simulink model "FPGA_UART"  (R2024a)
settings: Solver=FixedStepDiscrete  StartTime=0.0  StopTime=0.05  RelTol=1e-3
values from neighbouring files (symbols this model uses):
  Ts = 1/Fs    (= 7.50007500075e-06)    [new_generation_coeff.m]    (also in simon_test.m; simple_fft_test.m = 1/F; testPSD_c2d.m; testPSD_simulink.m)
libraries: hdlsllib x78, simulink_extras x12, simulink x5
(part 1 of 2)
settings Model: SimulationMode=accelerator  Creator=Simon  LastModifiedBy=Simon

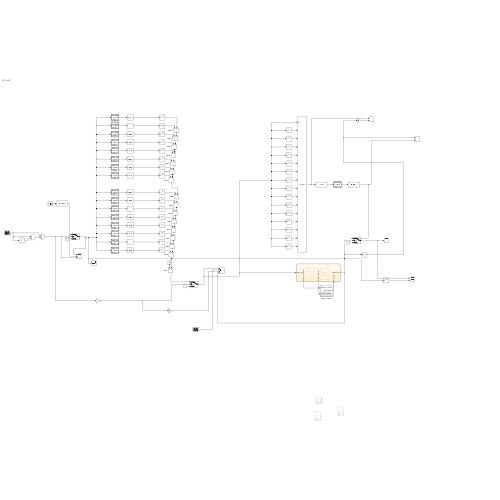
[thumbnail: Simulink's stored preview of the top-level diagram]
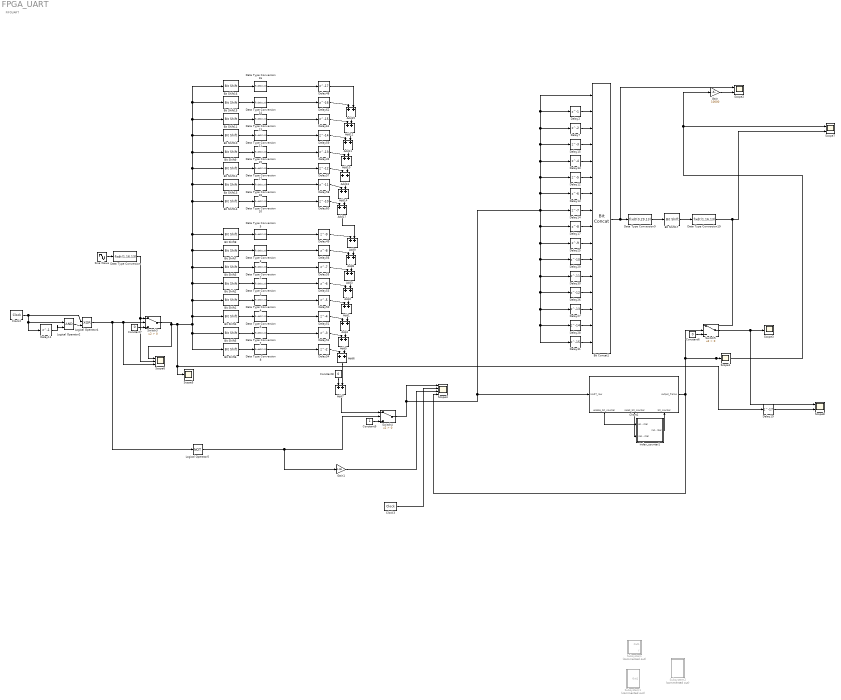
== system FPGA_UART ==
  note: FIFOUART
  Add{1..15,17} (16 alike) : Sum  OutDataTypeStr=fixdt(0,1,0)
  Bit Concat1 : hdlsllib/Logic and Bit Operations/Bit Concat  numInputs=16
  Bit Shift1 : hdlsllib/Logic and Bit Operations/Bit Shift  mode=Shift Left Logical  N=10
  Bit Shift10 : hdlsllib/Logic and Bit Operations/Bit Shift  mode=Shift Left Logical  N=1
  Bit Shift11 : hdlsllib/Logic and Bit Operations/Bit Shift  mode=Shift Right Logical  N=0
  Bit Shift12 : hdlsllib/Logic and Bit Operations/Bit Shift  mode=Shift Left Logical  N=3
  Bit Shift13 : hdlsllib/Logic and Bit Operations/Bit Shift  mode=Shift Left Logical  N=4
  Bit Shift14 : hdlsllib/Logic and Bit Operations/Bit Shift  mode=Shift Left Logical  N=5
  Bit Shift15 : hdlsllib/Logic and Bit Operations/Bit Shift  mode=Shift Right Logical  N=1
  Bit Shift16 : hdlsllib/Logic and Bit Operations/Bit Shift  mode=Shift Right Logical  N=2
  Bit Shift17 : hdlsllib/Logic and Bit Operations/Bit Shift  mode=Shift Right Logical  N=13
  Bit Shift2 : hdlsllib/Logic and Bit Operations/Bit Shift  mode=Shift Left Logical  N=9
  Bit Shift3 : hdlsllib/Logic and Bit Operations/Bit Shift  mode=Shift Left Logical  N=8
  Bit Shift4 : hdlsllib/Logic and Bit Operations/Bit Shift  mode=Shift Left Logical  N=11
  Bit Shift5 : hdlsllib/Logic and Bit Operations/Bit Shift  mode=Shift Left Logical  N=12
  Bit Shift6 : hdlsllib/Logic and Bit Operations/Bit Shift  mode=Shift Left Logical  N=13
  Bit Shift7 : hdlsllib/Logic and Bit Operations/Bit Shift  mode=Shift Left Logical  N=7
  Bit Shift8 : hdlsllib/Logic and Bit Operations/Bit Shift  mode=Shift Left Logical  N=6
  Bit Shift9 : hdlsllib/Logic and Bit Operations/Bit Shift  mode=Shift Left Logical  N=2
  Chart1 : Stateflow chart  TreatAsAtomicUnit=on
      settings: PortSchema="{\"entries\":[{\"content\":{\"sides\":[{\"content\":{\"connectorIds\":[\"In2\"]},\"type\":\"ConnectorPlacement.EquallySpacedRectSide\",\"uuid\":\"2ee02e2e-a069-4e33-9774-57cdf73b0390\"},{\"content\":{\"connectorIds\":[\"Out1\"],\"side\":\"RIGHT\"},\"type\":\"ConnectorPlacement.EquallySpacedRectSide\",\"uuid\":\"21aeb1e6-6c65-4c00-a9b7-a995856e37fb\"},{\"content\":{\"side\":\"TOP\"},\"type\":\"ConnectorPlacement.EquallySpacedRectSide\",\"uuid\":\"d38f9540-57bf-4030-828c-0c58160bc96c\"},{\"content\":{\"connectorIds\":[\"Out2\",\"Out3\",\"In1\"],\"side\":\"BOTTOM\"},\"type\":\"ConnectorPlacement.EquallySpacedRectSide\",\"uuid\":\"4fe203c5-9b79-43fe-8008-8789174ca3d6\"}]},\"type\":\"ConnectorPlacement.EquallySpacedConnector\",\"uuid\":\"11cdfd4e-ecb7-4173-8729-c2a9bb2b5432\"}],\"packageUris\":[\"http://schema.mathworks.com/mf0/Connector/R2020b\"],\"version\":\"1.0\"}"
  Clock2 : simulink_extras/Flip Flops/Clock  period=Ts*18
  Clock3 : simulink_extras/Flip Flops/Clock  period=Ts
  Constant6 : Constant  Value=0  OutDataTypeStr=fixdt(0,4,0)  SampleTime=Ts
  Constant7 : Constant  Value=0  OutDataTypeStr=fixdt(0,4,0)  SampleTime=Ts
  Constant8 : Constant  Value=0  OutDataTypeStr=fixdt(0,4,0)  SampleTime=Ts
  Constant9 : Constant  OutDataTypeStr=fixdt(0,4,0)  SampleTime=Ts
  Data Type Conversion : DataTypeConversion  OutDataTypeStr=fixdt(1,16,13)  SaturateOnIntegerOverflow=off  RndMeth=Floor
  Data Type Conversion{1..8,10..11,13..18} (16 alike) : DataTypeConversion  OutDataTypeStr=fixdt(0,1,0)  SaturateOnIntegerOverflow=off  RndMeth=Floor
  Data Type Conversion19 : DataTypeConversion  OutDataTypeStr=fixdt(1,16,13)  SaturateOnIntegerOverflow=off  RndMeth=Floor
  Data Type Conversion9 : DataTypeConversion  OutDataTypeStr=fixdt(0,29,13)  SaturateOnIntegerOverflow=off  RndMeth=Floor
  Delay11 : Delay  DelayLength=1  InitialCondition=0  SampleTime=Ts
  Delay12 : Delay  DelayLength=5  InitialCondition=0  SampleTime=Ts
  Delay13 : Delay  DelayLength=6  InitialCondition=0  SampleTime=Ts
  Delay14 : Delay  DelayLength=7  InitialCondition=0  SampleTime=Ts
  Delay15 : Delay  DelayLength=3  InitialCondition=0  SampleTime=Ts
  Delay17 : Delay  DelayLength=8  InitialCondition=0  SampleTime=Ts
  Delay19 : Delay  DelayLength=17  InitialCondition=0
  Delay2 : Delay  DelayLength=1  InitialCondition=0  SampleTime=Ts
  Delay25 : Delay  DelayLength=9  InitialCondition=0  SampleTime=Ts
  Delay26 : Delay  DelayLength=12  InitialCondition=0  SampleTime=Ts
  Delay27 : Delay  DelayLength=13  InitialCondition=0  SampleTime=Ts
  Delay28 : Delay  DelayLength=14  InitialCondition=0  SampleTime=Ts
  Delay29 : Delay  DelayLength=10  InitialCondition=0  SampleTime=Ts
  Delay30 : Delay  DelayLength=11  InitialCondition=0  SampleTime=Ts
  Delay31 : Delay  DelayLength=15  InitialCondition=0  SampleTime=Ts
  Delay32 : Delay  DelayLength=13  InitialCondition=0  SampleTime=Ts
  Delay33 : Delay  DelayLength=4  InitialCondition=0  SampleTime=Ts
  Delay48 : Delay  DelayLength=17  InitialCondition=0  SampleTime=Ts
  Delay49 : Delay  DelayLength=9  InitialCondition=0  SampleTime=Ts
  Delay50 : Delay  DelayLength=5  InitialCondition=0  SampleTime=Ts
  Delay51 : Delay  DelayLength=4  InitialCondition=0  SampleTime=Ts
  Delay52 : Delay  DelayLength=3  InitialCondition=0  SampleTime=Ts
  Delay53 : Delay  DelayLength=6  InitialCondition=0  SampleTime=Ts
  Delay54 : Delay  InitialCondition=0  SampleTime=Ts
  Delay55 : Delay  DelayLength=7  InitialCondition=0  SampleTime=Ts
  Delay56 : Delay  DelayLength=8  InitialCondition=0  SampleTime=Ts
  Delay57 : Delay  DelayLength=12  InitialCondition=0  SampleTime=Ts
  Delay58 : Delay  DelayLength=11  InitialCondition=0  SampleTime=Ts
  Delay59 : Delay  DelayLength=14  InitialCondition=0  SampleTime=Ts
  Delay60 : Delay  DelayLength=10  InitialCondition=0  SampleTime=Ts
  Delay61 : Delay  DelayLength=15  InitialCondition=0  SampleTime=Ts
  Delay62 : Delay  DelayLength=16  InitialCondition=0  SampleTime=Ts
  Delay7 : Delay  InitialCondition=0  SampleTime=Ts
  Gain : Gain  Gain=10000
  Gain1 : Gain  Gain=1.05
  Logical Operator2 : Logic  IconShape=distinctive  AllPortsSameDT=off  OutDataTypeStr=boolean
  Logical Operator4 : Logic  Operator=XOR  IconShape=distinctive  AllPortsSameDT=off  OutDataTypeStr=boolean
  Logical Operator5 : Logic  Operator=NOT  IconShape=distinctive  AllPortsSameDT=off  OutDataTypeStr=boolean
  Scope1 : Scope
  Scope2 : Scope  NumInputPorts=2
  Scope3 : Scope
  Scope4 : Scope  NumInputPorts=4
  Scope5 : Scope
  Scope6 : Scope  NumInputPorts=3
  Scope7 : Scope  NumInputPorts=2
  Scope8 : Scope  NumInputPorts=2
  Sine Wave : Sin  Amplitude=2  Frequency=1000  SampleTime=Ts*18
  Subsystem : Subsystem  Commented=on
  Subsystem1 : Subsystem  Commented=on
  Subsystem2 : Subsystem  Commented=on
  Switch3 : Switch  Criteria=u2 > Threshold  SaturateOnIntegerOverflow=off  InputSameDT=off  OutDataTypeStr=Inherit: Same as first input
  Switch4 : Switch  Criteria=u2 > Threshold  OutDataTypeStr=fixdt(0,1,0)  SaturateOnIntegerOverflow=off  InputSameDT=off
  Switch5 : Switch  Criteria=u2 > Threshold  SaturateOnIntegerOverflow=off  InputSameDT=off  OutDataTypeStr=Inherit: Same as first input
  index_counter1 : Subsystem
  wires:
  Delay19/1 -> Scope8/2
  Switch5/1 -> Scope8/1, Scope3/1
  Data Type Conversion/1 -> Scope6/2, Switch3/1
  Data Type Conversion9/1 -> Bit Shift17/1
  Bit Shift17/1 -> Data Type Conversion19/1
  Delay26/1 -> Bit Concat1/13
  Delay30/1 -> Bit Concat1/12
  Delay33/1 -> Bit Concat1/5
  Delay27/1 -> Bit Concat1/14
  Delay29/1 -> Bit Concat1/11
  Delay28/1 -> Bit Concat1/15
  Delay17/1 -> Bit Concat1/9
  Delay14/1 -> Bit Concat1/8
  Delay13/1 -> Bit Concat1/7
  Delay31/1 -> Bit Concat1/16
  Delay15/1 -> Bit Concat1/4
  Delay7/1 -> Bit Concat1/3
  Delay12/1 -> Bit Concat1/6
  Switch4/1 -> Delay31/1, Delay28/1, Delay27/1, Delay26/1, Delay30/1, Delay29/1, Delay25/1, Delay17/1, Delay14/1, Delay2/1, Bit Concat1/1, Delay7/1, Delay15/1, Delay33/1, Delay12/1, Delay13/1, Chart1/2(UART_raw), Scope4/1
  Delay25/1 -> Bit Concat1/10
  Delay2/1 -> Bit Concat1/2
  Gain/1 -> Scope2/2
  Data Type Conversion19/1 -> Scope7/2, Switch5/1
  Bit Shift6/1 -> Data Type Conversion8/1
  Add14/1 -> Add17/2
  Add17/1 -> Add9/2
  Delay60/1 -> Add17/1
  Add13/1 -> Add14/2
  Delay57/1 -> Add13/1
  Delay32/1 -> Add10/1
  Bit Shift9/1 -> Data Type Conversion15/1
  Bit Shift13/1 -> Data Type Conversion18/1
  Delay58/1 -> Add14/1
  Data Type Conversion17/1 -> Delay57/1
  Bit Shift12/1 -> Data Type Conversion17/1
  Data Type Conversion18/1 -> Delay58/1
  Data Type Conversion15/1 -> Delay32/1
  Data Type Conversion11/1 -> Delay59/1
  Bit Shift10/1 -> Data Type Conversion11/1
  Add10/1 -> Add13/2
  Delay61/1 -> Add12/1
  Bit Shift11/1 -> Data Type Conversion13/1
  Data Type Conversion13/1 -> Delay61/1
  Data Type Conversion14/1 -> Delay62/1
  Bit Shift15/1 -> Data Type Conversion14/1
  Delay62/1 -> Add15/1
  Bit Shift16/1 -> Data Type Conversion16/1
  Data Type Conversion16/1 -> Delay48/1
  Add11/1 -> Add10/2
  Delay59/1 -> Add11/1
  Add12/1 -> Add11/2
  Add15/1 -> Add12/2
  Switch3/1 -> Delay19/1, Scope5/1, Bit Shift4/1, Bit Shift1/1, Bit Shift2/1, Bit Shift3/1, Bit Shift7/1, Bit Shift8/1, Bit Shift14/1, Bit Shift13/1, Bit Shift12/1, Bit Shift9/1, Bit Shift10/1, Bit Shift11/1, Bit Shift15/1, Bit Shift16/1, Bit Shift6/1, Bit Shift5/1, Scope6/1
  Delay48/1 -> Add15/2
  Add9/1 -> Add8/2
  Bit Shift14/1 -> Data Type Conversion10/1
  Data Type Conversion10/1 -> Delay60/1
  Add8/1 -> Add3/2
  Add3/1 -> Add2/2
  Delay53/1 -> Add2/1
  Add2/1 -> Add1/2
  Data Type Conversion5/1 -> Delay49/1
  Bit Shift8/1 -> Data Type Conversion5/1
  Delay49/1 -> Add9/1
  Delay56/1 -> Add8/1
  Bit Shift7/1 -> Data Type Conversion3/1
  Data Type Conversion3/1 -> Delay56/1
  Data Type Conversion2/1 -> Delay55/1
  Bit Shift3/1 -> Data Type Conversion2/1
  Delay55/1 -> Add3/1
  Add1/1 -> Add4/2
  Bit Shift2/1 -> Data Type Conversion1/1
  Data Type Conversion1/1 -> Delay53/1
  Data Type Conversion4/1 -> Delay50/1
  Add6/1 -> Add7/2
  Data Type Conversion7/1 -> Delay52/1
  Bit Shift4/1 -> Data Type Conversion6/1
  Delay11/1 -> Logical Operator2/2
  Chart1/3(reset_bit_counter) -> index_counter1/2(reset_bit_counter)
  Constant9/1 -> Switch4/3
  Logical Operator2/1 -> Logical Operator4/2
  Constant7/1 -> Switch3/3
  Delay54/1 -> Add6/1
  Data Type Conversion6/1 -> Delay51/1
  Add5/1 -> Add6/2
  Gain1/1 -> Scope4/3
  Data Type Conversion8/1 -> Delay54/1
  Delay52/1 -> Add5/1
  Bit Shift5/1 -> Data Type Conversion7/1
  Clock3/1 -> Scope4/2
  Bit Shift1/1 -> Data Type Conversion4/1
  Sine Wave/1 -> Data Type Conversion/1
  Add7/1 -> Switch4/1
  Logical Operator5/1 -> Gain1/1, Switch4/2
  Delay50/1 -> Add1/1
  Logical Operator4/1 -> Logical Operator5/1, Scope6/3, Switch3/2
  Delay51/1 -> Add4/1
  index_counter1/1(index_counter) -> Chart1/1(bit_counter)
  Chart1/2(enable_bit_counter) -> index_counter1/1(enable_bit_counter)
  Chart1/1(output_frame) -> Scope1/1, Scope7/1, Gain/1, Switch5/2, Scope4/4
  Constant8/1 -> Add7/1
  Clock2/1 -> Delay11/1, Logical Operator2/1, Logical Operator4/1
  Add4/1 -> Add5/2
  Bit Concat1/1 -> Data Type Conversion9/1, Scope2/1
  Constant6/1 -> Switch5/3

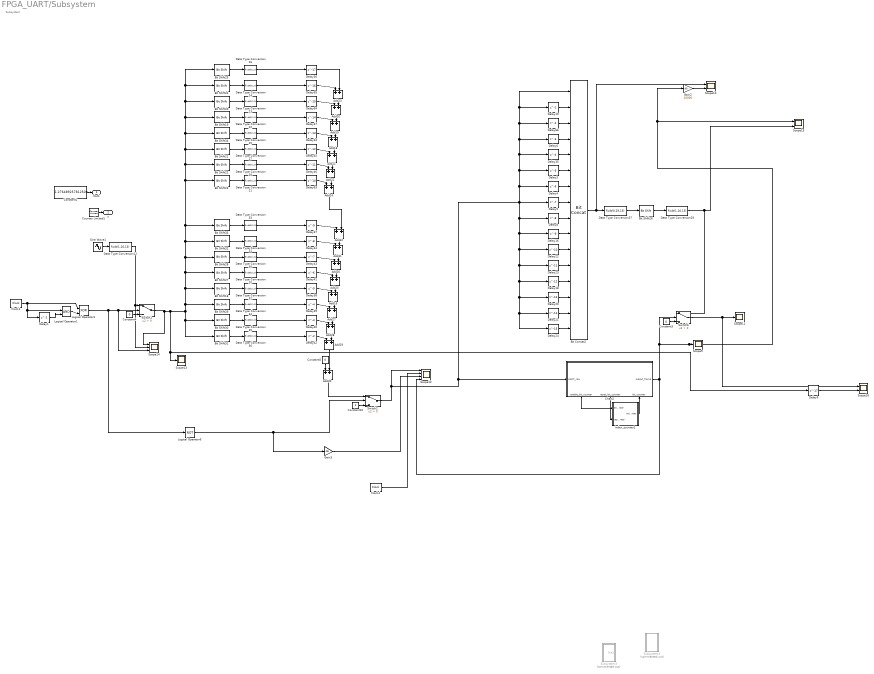
== system FPGA_UART/Subsystem ==
  note: Subsystem
  Add{16,18..32} (16 alike) : Sum  OutDataTypeStr=fixdt(0,1,0)
  Bit Concat2 : hdlsllib/Logic and Bit Operations/Bit Concat  numInputs=16
  Bit Shift18 : hdlsllib/Logic and Bit Operations/Bit Shift  mode=Shift Left Logical  N=10
  Bit Shift19 : hdlsllib/Logic and Bit Operations/Bit Shift  mode=Shift Left Logical  N=1
  Bit Shift20 : hdlsllib/Logic and Bit Operations/Bit Shift  mode=Shift Right Logical  N=0
  Bit Shift21 : hdlsllib/Logic and Bit Operations/Bit Shift  mode=Shift Left Logical  N=3
  Bit Shift22 : hdlsllib/Logic and Bit Operations/Bit Shift  mode=Shift Left Logical  N=4
  Bit Shift23 : hdlsllib/Logic and Bit Operations/Bit Shift  mode=Shift Left Logical  N=5
  Bit Shift24 : hdlsllib/Logic and Bit Operations/Bit Shift  mode=Shift Right Logical  N=1
  Bit Shift25 : hdlsllib/Logic and Bit Operations/Bit Shift  mode=Shift Right Logical  N=2
  Bit Shift26 : hdlsllib/Logic and Bit Operations/Bit Shift  mode=Shift Right Logical  N=13
  Bit Shift27 : hdlsllib/Logic and Bit Operations/Bit Shift  mode=Shift Left Logical  N=9
  Bit Shift28 : hdlsllib/Logic and Bit Operations/Bit Shift  mode=Shift Left Logical  N=8
  Bit Shift29 : hdlsllib/Logic and Bit Operations/Bit Shift  mode=Shift Left Logical  N=11
  Bit Shift30 : hdlsllib/Logic and Bit Operations/Bit Shift  mode=Shift Left Logical  N=12
  Bit Shift31 : hdlsllib/Logic and Bit Operations/Bit Shift  mode=Shift Left Logical  N=13
  Bit Shift32 : hdlsllib/Logic and Bit Operations/Bit Shift  mode=Shift Left Logical  N=7
  Bit Shift33 : hdlsllib/Logic and Bit Operations/Bit Shift  mode=Shift Left Logical  N=6
  Bit Shift34 : hdlsllib/Logic and Bit Operations/Bit Shift  mode=Shift Left Logical  N=2
  Chart2 : Stateflow chart  TreatAsAtomicUnit=on
      settings: PortSchema="{\"entries\":[{\"content\":{\"sides\":[{\"content\":{\"connectorIds\":[\"In2\"]},\"type\":\"ConnectorPlacement.EquallySpacedRectSide\",\"uuid\":\"2ee02e2e-a069-4e33-9774-57cdf73b0390\"},{\"content\":{\"connectorIds\":[\"Out1\"],\"side\":\"RIGHT\"},\"type\":\"ConnectorPlacement.EquallySpacedRectSide\",\"uuid\":\"21aeb1e6-6c65-4c00-a9b7-a995856e37fb\"},{\"content\":{\"side\":\"TOP\"},\"type\":\"ConnectorPlacement.EquallySpacedRectSide\",\"uuid\":\"d38f9540-57bf-4030-828c-0c58160bc96c\"},{\"content\":{\"connectorIds\":[\"Out2\",\"Out3\",\"In1\"],\"side\":\"BOTTOM\"},\"type\":\"ConnectorPlacement.EquallySpacedRectSide\",\"uuid\":\"4fe203c5-9b79-43fe-8008-8789174ca3d6\"}]},\"type\":\"ConnectorPlacement.EquallySpacedConnector\",\"uuid\":\"11cdfd4e-ecb7-4173-8729-c2a9bb2b5432\"}],\"packageUris\":[\"http://schema.mathworks.com/mf0/Connector/R2020b\"],\"version\":\"1.0\"}"
  Clock1 : simulink_extras/Flip Flops/Clock  period=Ts*18
  Clock4 : simulink_extras/Flip Flops/Clock  period=Ts
  Constant1 : Constant  Value=1.276489257812500  OutDataTypeStr=fixdt(1,16,13)  SampleTime=Ts
  Constant10 : Constant  OutDataTypeStr=fixdt(0,4,0)  SampleTime=Ts
  Constant3 : Constant  Value=0  OutDataTypeStr=fixdt(0,4,0)  SampleTime=Ts
  Constant4 : Constant  Value=0  OutDataTypeStr=fixdt(0,4,0)  SampleTime=Ts
  Constant5 : Constant  Value=0  OutDataTypeStr=fixdt(0,4,0)  SampleTime=Ts
  Counter Limited1 : simulink/Sources/Counter Limited  uplimit=32  tsamp=Ts*18
  Data Type Conversion12 : DataTypeConversion  OutDataTypeStr=fixdt(1,16,13)  SaturateOnIntegerOverflow=off  RndMeth=Floor
  Data Type Conversion{20..28,30..36} (16 alike) : DataTypeConversion  OutDataTypeStr=fixdt(0,1,0)  SaturateOnIntegerOverflow=off  RndMeth=Floor
  Data Type Conversion29 : DataTypeConversion  OutDataTypeStr=fixdt(1,16,13)  SaturateOnIntegerOverflow=off  RndMeth=Floor
  Data Type Conversion37 : DataTypeConversion  OutDataTypeStr=fixdt(0,29,13)  SaturateOnIntegerOverflow=off  RndMeth=Floor
  Delay1 : Delay  DelayLength=1  InitialCondition=0  SampleTime=Ts
  Delay10 : Delay  DelayLength=1  InitialCondition=0  SampleTime=Ts
  Delay16 : Delay  DelayLength=9  InitialCondition=0  SampleTime=Ts
  Delay18 : Delay  DelayLength=12  InitialCondition=0  SampleTime=Ts
  Delay20 : Delay  DelayLength=13  InitialCondition=0  SampleTime=Ts
  Delay21 : Delay  DelayLength=14  InitialCondition=0  SampleTime=Ts
  Delay22 : Delay  DelayLength=10  InitialCondition=0  SampleTime=Ts
  Delay23 : Delay  DelayLength=11  InitialCondition=0  SampleTime=Ts
  Delay24 : Delay  DelayLength=15  InitialCondition=0  SampleTime=Ts
  Delay3 : Delay  DelayLength=5  InitialCondition=0  SampleTime=Ts
  Delay34 : Delay  DelayLength=13  InitialCondition=0  SampleTime=Ts
  Delay35 : Delay  DelayLength=4  InitialCondition=0  SampleTime=Ts
  Delay36 : Delay  DelayLength=17  InitialCondition=0  SampleTime=Ts
  Delay37 : Delay  DelayLength=9  InitialCondition=0  SampleTime=Ts
  Delay38 : Delay  DelayLength=5  InitialCondition=0  SampleTime=Ts
  Delay39 : Delay  DelayLength=4  InitialCondition=0  SampleTime=Ts
  Delay4 : Delay  DelayLength=6  InitialCondition=0  SampleTime=Ts
  Delay40 : Delay  DelayLength=3  InitialCondition=0  SampleTime=Ts
  Delay41 : Delay  DelayLength=6  InitialCondition=0  SampleTime=Ts
  Delay42 : Delay  InitialCondition=0  SampleTime=Ts
  Delay43 : Delay  DelayLength=7  InitialCondition=0  SampleTime=Ts
  Delay44 : Delay  DelayLength=8  InitialCondition=0  SampleTime=Ts
  Delay45 : Delay  DelayLength=12  InitialCondition=0  SampleTime=Ts
  Delay46 : Delay  DelayLength=11  InitialCondition=0  SampleTime=Ts
  Delay47 : Delay  DelayLength=14  InitialCondition=0  SampleTime=Ts
  Delay5 : Delay  DelayLength=7  InitialCondition=0  SampleTime=Ts
  Delay6 : Delay  DelayLength=3  InitialCondition=0  SampleTime=Ts
  Delay63 : Delay  DelayLength=10  InitialCondition=0  SampleTime=Ts
  Delay64 : Delay  DelayLength=15  InitialCondition=0  SampleTime=Ts
  Delay65 : Delay  DelayLength=16  InitialCondition=0  SampleTime=Ts
  Delay66 : Delay  InitialCondition=0  SampleTime=Ts
  Delay8 : Delay  DelayLength=8  InitialCondition=0  SampleTime=Ts
  Delay9 : Delay  DelayLength=17  InitialCondition=0
  Gain2 : Gain  Gain=10000
  Gain3 : Gain  Gain=1.05
  Logical Operator1 : Logic  IconShape=distinctive  AllPortsSameDT=off  OutDataTypeStr=boolean
  Logical Operator3 : Logic  Operator=XOR  IconShape=distinctive  AllPortsSameDT=off  OutDataTypeStr=boolean
  Logical Operator6 : Logic  Operator=NOT  IconShape=distinctive  AllPortsSameDT=off  OutDataTypeStr=boolean
  Scope10 : Scope  NumInputPorts=2
  Scope11 : Scope
  Scope12 : Scope  NumInputPorts=4
  Scope13 : Scope
  Scope14 : Scope  NumInputPorts=3
  Scope15 : Scope  NumInputPorts=2
  Scope16 : Scope  NumInputPorts=2
  Scope9 : Scope
  Sine Wave1 : Sin  Amplitude=2  Frequency=1000  SampleTime=Ts*18
  Subsystem3 : Subsystem  Commented=on
  Subsystem4 : Subsystem  Commented=on
  Switch1 : Switch  Criteria=u2 > Threshold  SaturateOnIntegerOverflow=off  InputSameDT=off  OutDataTypeStr=Inherit: Same as first input
  Switch2 : Switch  Criteria=u2 > Threshold  OutDataTypeStr=fixdt(0,1,0)  SaturateOnIntegerOverflow=off  InputSameDT=off
  Switch6 : Switch  Criteria=u2 > Threshold  SaturateOnIntegerOverflow=off  InputSameDT=off  OutDataTypeStr=Inherit: Same as first input
  index_counter2 : Subsystem
  Out1 : Outport
  y : Outport  Port=2
  wires:
  Add23/1 -> Add20/2
  Add27/1 -> Add28/2
  Switch2/1 -> Delay24/1, Delay21/1, Delay20/1, Delay18/1, Delay23/1, Delay22/1, Delay16/1, Delay8/1, Delay5/1, Delay10/1, Bit Concat2/1, Delay66/1, Delay6/1, Delay35/1, Delay3/1, Delay4/1, Chart2/2(UART_raw), Scope12/1
  Switch1/1 -> Delay9/1, Scope13/1, Bit Shift29/1, Bit Shift18/1, Bit Shift27/1, Bit Shift28/1, Bit Shift32/1, Bit Shift33/1, Bit Shift23/1, Bit Shift22/1, Bit Shift21/1, Bit Shift34/1, Bit Shift19/1, Bit Shift20/1, Bit Shift24/1, Bit Shift25/1, Bit Shift31/1, Bit Shift30/1, Scope14/1
  Add25/1 -> Add16/2
  Clock1/1 -> Delay1/1, Logical Operator1/1, Logical Operator3/1
  Delay66/1 -> Bit Concat2/3
  Logical Operator3/1 -> Logical Operator6/1, Scope14/3, Switch1/2
  Delay38/1 -> Add16/1
  Delay44/1 -> Add31/1
  Delay37/1 -> Add32/1
  Add30/1 -> Switch2/1
  Delay22/1 -> Bit Concat2/11
  Add21/1 -> Add22/2
  Clock4/1 -> Scope12/2
  Add31/1 -> Add26/2
  Delay65/1 -> Add23/1
  Bit Shift19/1 -> Data Type Conversion22/1
  Delay36/1 -> Add23/2
  Bit Shift21/1 -> Data Type Conversion27/1
  Constant4/1 -> Switch1/3
  Bit Shift23/1 -> Data Type Conversion21/1
  Delay42/1 -> Add29/1
  Data Type Conversion27/1 -> Delay45/1
  Delay35/1 -> Bit Concat2/5
  Data Type Conversion31/1 -> Delay44/1
  Add28/1 -> Add29/2
  Bit Shift33/1 -> Data Type Conversion33/1
  Add22/1 -> Add24/2
  Switch6/1 -> Scope16/1, Scope11/1
  Add20/1 -> Add19/2
  Data Type Conversion29/1 -> Scope15/2, Switch6/1
  Delay6/1 -> Bit Concat2/4
  Delay16/1 -> Bit Concat2/10
  Add24/1 -> Add32/2
  Bit Shift27/1 -> Data Type Conversion20/1
  Chart2/1(output_frame) -> Scope9/1, Scope15/1, Gain2/1, Switch6/2, Scope12/4
  Add32/1 -> Add31/2
  Delay47/1 -> Add19/1
  Gain3/1 -> Scope12/3
  Data Type Conversion21/1 -> Delay63/1
  Delay34/1 -> Add18/1
  Data Type Conversion23/1 -> Delay64/1
  Bit Shift20/1 -> Data Type Conversion23/1
  Add19/1 -> Add18/2
  Data Type Conversion22/1 -> Delay47/1
  Constant5/1 -> Add30/1
  Data Type Conversion24/1 -> Delay65/1
  Bit Shift34/1 -> Data Type Conversion25/1
  Add18/1 -> Add21/2
  Delay20/1 -> Bit Concat2/14
  Data Type Conversion25/1 -> Delay34/1
  Delay64/1 -> Add20/1
  Data Type Conversion26/1 -> Delay36/1
  Bit Shift24/1 -> Data Type Conversion24/1
  Data Type Conversion20/1 -> Delay41/1
  Delay43/1 -> Add26/1
  Delay41/1 -> Add25/1
  Bit Shift25/1 -> Data Type Conversion26/1
  Bit Shift32/1 -> Data Type Conversion31/1
  Constant3/1 -> Switch6/3
  Data Type Conversion12/1 -> Scope14/2, Switch1/1
  Data Type Conversion28/1 -> Delay46/1
  Constant1/1 -> Out1/1
  Bit Shift22/1 -> Data Type Conversion28/1
  Data Type Conversion30/1 -> Delay43/1
  Delay46/1 -> Add22/1
  Data Type Conversion33/1 -> Delay37/1
  Data Type Conversion34/1 -> Delay39/1
  Logical Operator1/1 -> Logical Operator3/2
  Bit Shift28/1 -> Data Type Conversion30/1
  Add16/1 -> Add27/2
  Delay24/1 -> Bit Concat2/16
  Delay5/1 -> Bit Concat2/8
  Data Type Conversion32/1 -> Delay38/1
  Delay18/1 -> Bit Concat2/13
  Bit Shift26/1 -> Data Type Conversion29/1
  Bit Shift31/1 -> Data Type Conversion36/1
  Data Type Conversion37/1 -> Bit Shift26/1
  Delay9/1 -> Scope16/2
  Sine Wave1/1 -> Data Type Conversion12/1
  Chart2/2(enable_bit_counter) -> index_counter2/1(enable_bit_counter)
  Delay21/1 -> Bit Concat2/15
  Delay8/1 -> Bit Concat2/9
  Delay1/1 -> Logical Operator1/2
  Delay4/1 -> Bit Concat2/7
  Delay23/1 -> Bit Concat2/12
  index_counter2/1(index_counter) -> Chart2/1(bit_counter)
  Chart2/3(reset_bit_counter) -> index_counter2/2(reset_bit_counter)
  Delay39/1 -> Add27/1
  Data Type Conversion35/1 -> Delay40/1
  Bit Concat2/1 -> Data Type Conversion37/1, Scope10/1
  Constant10/1 -> Switch2/3
  Logical Operator6/1 -> Gain3/1, Switch2/2
  Add29/1 -> Add30/2
  Delay3/1 -> Bit Concat2/6
  Bit Shift29/1 -> Data Type Conversion34/1
  Bit Shift30/1 -> Data Type Conversion35/1
  Data Type Conversion36/1 -> Delay42/1
  Bit Shift18/1 -> Data Type Conversion32/1
  Delay40/1 -> Add28/1
  Add26/1 -> Add25/2
  Counter Limited1/1 -> y/1
  Delay45/1 -> Add21/1
  Delay63/1 -> Add24/1
  Gain2/1 -> Scope10/2
  Delay10/1 -> Bit Concat2/2

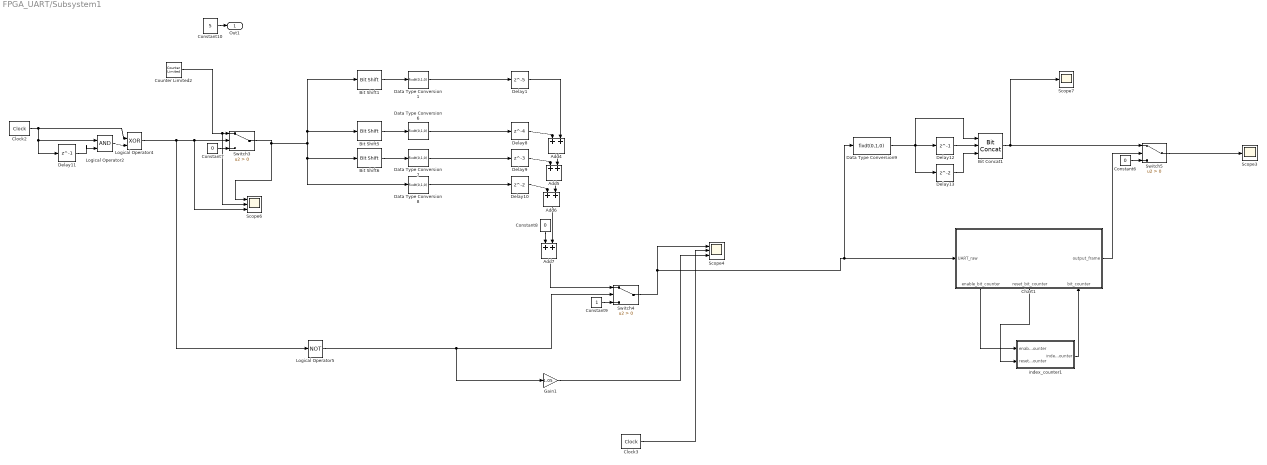
== system FPGA_UART/Subsystem1 ==
  Add{4..7} (4 alike) : Sum
  Bit Concat1 : hdlsllib/Logic and Bit Operations/Bit Concat  numInputs=3
  Bit Shift1 : hdlsllib/Logic and Bit Operations/Bit Shift  mode=Shift Right Logical  N=3
  Bit Shift5 : hdlsllib/Logic and Bit Operations/Bit Shift  mode=Shift Right Logical  N=2
  Bit Shift6 : hdlsllib/Logic and Bit Operations/Bit Shift  mode=Shift Right Logical  N=1
  Chart1 : Stateflow chart  TreatAsAtomicUnit=on
      settings: PortSchema="{\"entries\":[{\"content\":{\"sides\":[{\"content\":{\"connectorIds\":[\"In2\"]},\"type\":\"ConnectorPlacement.EquallySpacedRectSide\",\"uuid\":\"2ee02e2e-a069-4e33-9774-57cdf73b0390\"},{\"content\":{\"connectorIds\":[\"Out1\"],\"side\":\"RIGHT\"},\"type\":\"ConnectorPlacement.EquallySpacedRectSide\",\"uuid\":\"21aeb1e6-6c65-4c00-a9b7-a995856e37fb\"},{\"content\":{\"side\":\"TOP\"},\"type\":\"ConnectorPlacement.EquallySpacedRectSide\",\"uuid\":\"d38f9540-57bf-4030-828c-0c58160bc96c\"},{\"content\":{\"connectorIds\":[\"Out2\",\"Out3\",\"In1\"],\"side\":\"BOTTOM\"},\"type\":\"ConnectorPlacement.EquallySpacedRectSide\",\"uuid\":\"4fe203c5-9b79-43fe-8008-8789174ca3d6\"}]},\"type\":\"ConnectorPlacement.EquallySpacedConnector\",\"uuid\":\"11cdfd4e-ecb7-4173-8729-c2a9bb2b5432\"}],\"packageUris\":[\"http://schema.mathworks.com/mf0/Connector/R2020b\"],\"version\":\"1.0\"}"
  Clock2 : simulink_extras/Flip Flops/Clock  period=Ts*6
  Clock3 : simulink_extras/Flip Flops/Clock  period=Ts
  Constant10 : Constant  Value=5  OutDataTypeStr=fixdt(0,4,0)  SampleTime=Ts*5
  Constant6 : Constant  Value=0  OutDataTypeStr=fixdt(0,4,0)  SampleTime=Ts
  Constant7 : Constant  Value=0  OutDataTypeStr=fixdt(0,4,0)  SampleTime=Ts
  Constant8 : Constant  Value=0  OutDataTypeStr=fixdt(0,4,0)  SampleTime=Ts
  Constant9 : Constant  OutDataTypeStr=fixdt(0,4,0)  SampleTime=Ts
  Counter Limited2 : simulink/Sources/Counter Limited  uplimit=7  tsamp=Ts*6
  Data Type Conversion{1,6..8} (4 alike) : DataTypeConversion  OutDataTypeStr=fixdt(0,1,0)  SaturateOnIntegerOverflow=off  RndMeth=Floor
  Data Type Conversion9 : DataTypeConversion  OutDataTypeStr=fixdt(0,1,0)  RndMeth=Floor
  Delay1 : Delay  DelayLength=5  InitialCondition=0  SampleTime=Ts
  Delay10 : Delay  InitialCondition=0  SampleTime=Ts
  Delay11 : Delay  DelayLength=1  InitialCondition=0  SampleTime=Ts
  Delay12 : Delay  DelayLength=1  InitialCondition=0  SampleTime=Ts
  Delay13 : Delay  InitialCondition=0  SampleTime=Ts
  Delay8 : Delay  DelayLength=4  InitialCondition=0  SampleTime=Ts
  Delay9 : Delay  DelayLength=3  InitialCondition=0  SampleTime=Ts
  Gain1 : Gain  Gain=1.05
  Logical Operator2 : Logic  IconShape=distinctive  AllPortsSameDT=off  OutDataTypeStr=boolean
  Logical Operator4 : Logic  Operator=XOR  IconShape=distinctive  AllPortsSameDT=off  OutDataTypeStr=boolean
  Logical Operator5 : Logic  Operator=NOT  IconShape=distinctive  AllPortsSameDT=off  OutDataTypeStr=boolean
  Scope3 : Scope
  Scope4 : Scope  NumInputPorts=3
  Scope6 : Scope  NumInputPorts=3
  Scope7 : Scope
  Switch3 : Switch  Criteria=u2 > Threshold  SaturateOnIntegerOverflow=off  InputSameDT=off
  Switch4 : Switch  Criteria=u2 > Threshold  SaturateOnIntegerOverflow=off  InputSameDT=off
  Switch5 : Switch  Criteria=u2 > Threshold  OutDataTypeStr=fixdt(0,3,0)  SaturateOnIntegerOverflow=off  InputSameDT=off
  index_counter1 : Subsystem
  Out1 : Outport
  wires:
  Add6/1 -> Add7/2
  Data Type Conversion7/1 -> Delay9/1
  Bit Shift5/1 -> Data Type Conversion6/1
  Delay11/1 -> Logical Operator2/2
  Chart1/3(reset_bit_counter) -> index_counter1/2(reset_bit_counter)
  Constant9/1 -> Switch4/3
  Logical Operator2/1 -> Logical Operator4/2
  Constant7/1 -> Switch3/3
  Delay10/1 -> Add6/1
  Data Type Conversion6/1 -> Delay8/1
  Delay12/1 -> Bit Concat1/2
  Add5/1 -> Add6/2
  Gain1/1 -> Scope4/3
  Switch5/1 -> Scope3/1
  Data Type Conversion8/1 -> Delay10/1
  Delay9/1 -> Add5/1
  Delay13/1 -> Bit Concat1/3
  Bit Shift6/1 -> Data Type Conversion7/1
  Clock3/1 -> Scope4/2
  Counter Limited2/1 -> Switch3/1, Scope6/2
  Add7/1 -> Switch4/1
  Constant10/1 -> Out1/1
  Logical Operator5/1 -> Switch4/2, Gain1/1
  Logical Operator4/1 -> Switch3/2, Scope6/3, Logical Operator5/1
  Data Type Conversion9/1 -> Delay12/1, Delay13/1, Bit Concat1/1
  Delay8/1 -> Add4/1
  index_counter1/1(index_counter) -> Chart1/1(bit_counter)
  Chart1/2(enable_bit_counter) -> index_counter1/1(enable_bit_counter)
  Switch4/1 -> Scope4/1, Data Type Conversion9/1, Chart1/2(UART_raw)
  Chart1/1(output_frame) -> Switch5/2
  Constant8/1 -> Add7/1
  Clock2/1 -> Logical Operator4/1, Logical Operator2/1, Delay11/1
  Add4/1 -> Add5/2
  Bit Concat1/1 -> Scope7/1, Switch5/1
  Constant6/1 -> Switch5/3
  Delay1/1 -> Add4/2
  Switch3/1 -> Scope6/1, Bit Shift6/1, Data Type Conversion8/1, Bit Shift1/1, Bit Shift5/1
  Data Type Conversion1/1 -> Delay1/1
  Bit Shift1/1 -> Data Type Conversion1/1

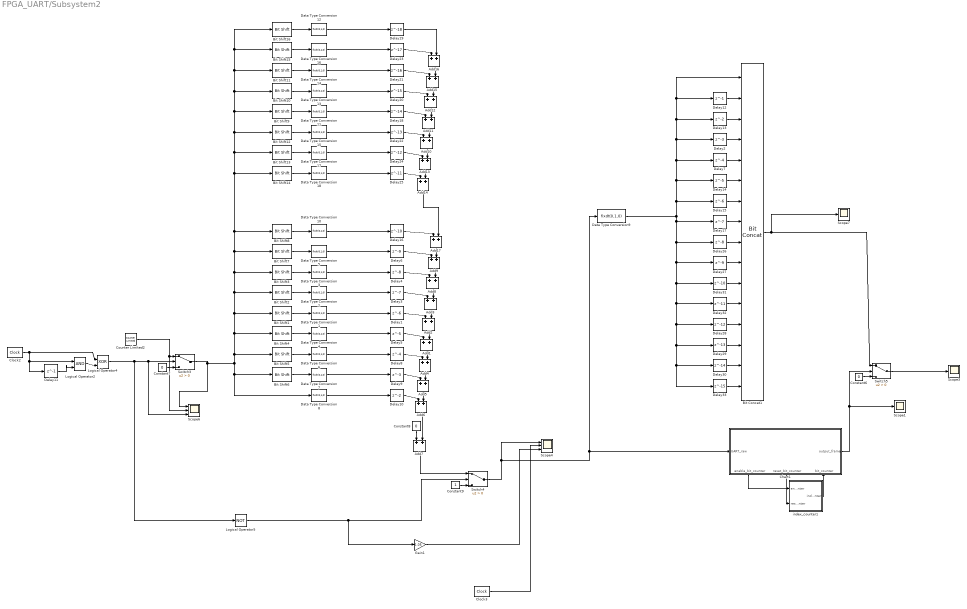
== system FPGA_UART/Subsystem2 ==
  Add{1..17} (17 alike) : Sum
  Bit Concat1 : hdlsllib/Logic and Bit Operations/Bit Concat  numInputs=16
  Bit Shift1 : hdlsllib/Logic and Bit Operations/Bit Shift  mode=Shift Right Logical  N=4
  Bit Shift10 : hdlsllib/Logic and Bit Operations/Bit Shift  mode=Shift Right Logical  N=13
  Bit Shift11 : hdlsllib/Logic and Bit Operations/Bit Shift  mode=Shift Right Logical  N=14
  Bit Shift12 : hdlsllib/Logic and Bit Operations/Bit Shift  mode=Shift Right Logical  N=11
  Bit Shift13 : hdlsllib/Logic and Bit Operations/Bit Shift  mode=Shift Right Logical  N=10
  Bit Shift14 : hdlsllib/Logic and Bit Operations/Bit Shift  mode=Shift Right Logical  N=9
  Bit Shift15 : hdlsllib/Logic and Bit Operations/Bit Shift  mode=Shift Right Logical  N=15
  Bit Shift16 : hdlsllib/Logic and Bit Operations/Bit Shift  mode=Shift Right Logical  N=16
  Bit Shift2 : hdlsllib/Logic and Bit Operations/Bit Shift  mode=Shift Right Logical  N=5
  Bit Shift3 : hdlsllib/Logic and Bit Operations/Bit Shift  mode=Shift Right Logical  N=6
  Bit Shift4 : hdlsllib/Logic and Bit Operations/Bit Shift  mode=Shift Right Logical  N=3
  Bit Shift5 : hdlsllib/Logic and Bit Operations/Bit Shift  mode=Shift Right Logical  N=2
  Bit Shift6 : hdlsllib/Logic and Bit Operations/Bit Shift  mode=Shift Right Logical  N=1
  Bit Shift7 : hdlsllib/Logic and Bit Operations/Bit Shift  mode=Shift Right Logical  N=7
  Bit Shift8 : hdlsllib/Logic and Bit Operations/Bit Shift  mode=Shift Right Logical  N=8
  Bit Shift9 : hdlsllib/Logic and Bit Operations/Bit Shift  mode=Shift Right Logical  N=12
  Chart1 : Stateflow chart  TreatAsAtomicUnit=on
      settings: PortSchema="{\"entries\":[{\"content\":{\"sides\":[{\"content\":{\"connectorIds\":[\"In2\"]},\"type\":\"ConnectorPlacement.EquallySpacedRectSide\",\"uuid\":\"2ee02e2e-a069-4e33-9774-57cdf73b0390\"},{\"content\":{\"connectorIds\":[\"Out1\"],\"side\":\"RIGHT\"},\"type\":\"ConnectorPlacement.EquallySpacedRectSide\",\"uuid\":\"21aeb1e6-6c65-4c00-a9b7-a995856e37fb\"},{\"content\":{\"side\":\"TOP\"},\"type\":\"ConnectorPlacement.EquallySpacedRectSide\",\"uuid\":\"d38f9540-57bf-4030-828c-0c58160bc96c\"},{\"content\":{\"connectorIds\":[\"Out2\",\"Out3\",\"In1\"],\"side\":\"BOTTOM\"},\"type\":\"ConnectorPlacement.EquallySpacedRectSide\",\"uuid\":\"4fe203c5-9b79-43fe-8008-8789174ca3d6\"}]},\"type\":\"ConnectorPlacement.EquallySpacedConnector\",\"uuid\":\"11cdfd4e-ecb7-4173-8729-c2a9bb2b5432\"}],\"packageUris\":[\"http://schema.mathworks.com/mf0/Connector/R2020b\"],\"version\":\"1.0\"}"
  Clock2 : simulink_extras/Flip Flops/Clock  period=Ts*18
  Clock3 : simulink_extras/Flip Flops/Clock  period=Ts
  Constant6 : Constant  Value=0  OutDataTypeStr=fixdt(0,4,0)  SampleTime=Ts
  Constant7 : Constant  Value=0  OutDataTypeStr=fixdt(0,4,0)  SampleTime=Ts
  Constant8 : Constant  Value=0  OutDataTypeStr=fixdt(0,4,0)  SampleTime=Ts
  Constant9 : Constant  OutDataTypeStr=fixdt(0,4,0)  SampleTime=Ts
  Counter Limited2 : simulink/Sources/Counter Limited  uplimit=65535  tsamp=Ts*18
  Data Type Conversion{1..8,10..18} (17 alike) : DataTypeConversion  OutDataTypeStr=fixdt(0,1,0)  SaturateOnIntegerOverflow=off  RndMeth=Floor
  Data Type Conversion9 : DataTypeConversion  OutDataTypeStr=fixdt(0,1,0)  RndMeth=Floor
  Delay1 : Delay  DelayLength=6  InitialCondition=0  SampleTime=Ts
  Delay10 : Delay  InitialCondition=0  SampleTime=Ts
  Delay11 : Delay  DelayLength=1  InitialCondition=0  SampleTime=Ts
  Delay12 : Delay  DelayLength=1  InitialCondition=0  SampleTime=Ts
  Delay13 : Delay  InitialCondition=0  SampleTime=Ts
  Delay14 : Delay  DelayLength=5  InitialCondition=0  SampleTime=Ts
  Delay15 : Delay  DelayLength=6  InitialCondition=0  SampleTime=Ts
  Delay16 : Delay  DelayLength=10  InitialCondition=0  SampleTime=Ts
  Delay17 : Delay  DelayLength=7  InitialCondition=0  SampleTime=Ts
  Delay18 : Delay  DelayLength=14  InitialCondition=0  SampleTime=Ts
  Delay19 : Delay  DelayLength=18  InitialCondition=0  SampleTime=Ts
  Delay2 : Delay  DelayLength=3  InitialCondition=0  SampleTime=Ts
  Delay20 : Delay  DelayLength=15  InitialCondition=0  SampleTime=Ts
  Delay21 : Delay  DelayLength=16  InitialCondition=0  SampleTime=Ts
  Delay22 : Delay  DelayLength=13  InitialCondition=0  SampleTime=Ts
  Delay23 : Delay  DelayLength=17  InitialCondition=0  SampleTime=Ts
  Delay24 : Delay  DelayLength=12  InitialCondition=0  SampleTime=Ts
  Delay25 : Delay  DelayLength=11  InitialCondition=0  SampleTime=Ts
  Delay26 : Delay  DelayLength=8  InitialCondition=0  SampleTime=Ts
  Delay27 : Delay  DelayLength=9  InitialCondition=0  SampleTime=Ts
  Delay28 : Delay  DelayLength=12  InitialCondition=0  SampleTime=Ts
  Delay29 : Delay  DelayLength=13  InitialCondition=0  SampleTime=Ts
  Delay3 : Delay  DelayLength=7  InitialCondition=0  SampleTime=Ts
  Delay30 : Delay  DelayLength=14  InitialCondition=0  SampleTime=Ts
  Delay31 : Delay  DelayLength=10  InitialCondition=0  SampleTime=Ts
  Delay32 : Delay  DelayLength=11  InitialCondition=0  SampleTime=Ts
  Delay33 : Delay  DelayLength=15  InitialCondition=0  SampleTime=Ts
  Delay4 : Delay  DelayLength=8  InitialCondition=0  SampleTime=Ts
  Delay5 : Delay  DelayLength=5  InitialCondition=0  SampleTime=Ts
  Delay6 : Delay  DelayLength=9  InitialCondition=0  SampleTime=Ts
  Delay7 : Delay  DelayLength=4  InitialCondition=0  SampleTime=Ts
  Delay8 : Delay  DelayLength=4  InitialCondition=0  SampleTime=Ts
  Delay9 : Delay  DelayLength=3  InitialCondition=0  SampleTime=Ts
  Gain1 : Gain  Gain=1.05
  Logical Operator2 : Logic  IconShape=distinctive  AllPortsSameDT=off  OutDataTypeStr=boolean
  Logical Operator4 : Logic  Operator=XOR  IconShape=distinctive  AllPortsSameDT=off  OutDataTypeStr=boolean
  Logical Operator5 : Logic  Operator=NOT  IconShape=distinctive  AllPortsSameDT=off  OutDataTypeStr=boolean
  Scope1 : Scope
  Scope3 : Scope
  Scope4 : Scope  NumInputPorts=3
  Scope6 : Scope  NumInputPorts=3
  Scope7 : Scope
  Switch3 : Switch  Criteria=u2 > Threshold  SaturateOnIntegerOverflow=off  InputSameDT=off
  Switch4 : Switch  Criteria=u2 > Threshold  SaturateOnIntegerOverflow=off  InputSameDT=off
  Switch5 : Switch  Criteria=u2 > Threshold  SaturateOnIntegerOverflow=off  InputSameDT=off  OutDataTypeStr=Inherit: Same as first input
  index_counter1 : Subsystem
  wires:
  Delay26/1 -> Bit Concat1/9
  Delay27/1 -> Bit Concat1/10
  Delay31/1 -> Bit Concat1/11
  Delay32/1 -> Bit Concat1/12
  Delay28/1 -> Bit Concat1/13
  Delay29/1 -> Bit Concat1/14
  Delay30/1 -> Bit Concat1/15
  Delay33/1 -> Bit Concat1/16
  Delay17/1 -> Bit Concat1/8
  Delay15/1 -> Bit Concat1/7
  Delay14/1 -> Bit Concat1/6
  Delay7/1 -> Bit Concat1/5
  Delay2/1 -> Bit Concat1/4
  Delay13/1 -> Bit Concat1/3
  Delay12/1 -> Bit Concat1/2
  Add14/1 -> Add17/2
  Add17/1 -> Add9/2
  Delay16/1 -> Add17/1
  Add13/1 -> Add14/2
  Delay24/1 -> Add13/1
  Delay22/1 -> Add10/1
  Bit Shift12/1 -> Data Type Conversion15/1
  Bit Shift14/1 -> Data Type Conversion18/1
  Delay25/1 -> Add14/1
  Data Type Conversion17/1 -> Delay24/1
  Bit Shift13/1 -> Data Type Conversion17/1
  Data Type Conversion18/1 -> Delay25/1
  Data Type Conversion15/1 -> Delay22/1
  Data Type Conversion11/1 -> Delay18/1
  Bit Shift9/1 -> Data Type Conversion11/1
  Add10/1 -> Add13/2
  Delay20/1 -> Add12/1
  Bit Shift10/1 -> Data Type Conversion13/1
  Data Type Conversion13/1 -> Delay20/1
  Data Type Conversion14/1 -> Delay21/1
  Bit Shift11/1 -> Data Type Conversion14/1
  Delay21/1 -> Add15/1
  Delay23/1 -> Add16/1
  Bit Shift15/1 -> Data Type Conversion16/1
  Data Type Conversion16/1 -> Delay23/1
  Add11/1 -> Add10/2
  Delay18/1 -> Add11/1
  Add12/1 -> Add11/2
  Add15/1 -> Add12/2
  Data Type Conversion12/1 -> Delay19/1
  Switch3/1 -> Scope6/1, Bit Shift6/1, Data Type Conversion8/1, Bit Shift5/1, Bit Shift4/1, Bit Shift1/1, Bit Shift2/1, Bit Shift3/1, Bit Shift7/1, Bit Shift8/1, Bit Shift14/1, Bit Shift13/1, Bit Shift12/1, Bit Shift9/1, Bit Shift10/1, Bit Shift11/1, Bit Shift16/1, Bit Shift15/1
  Bit Shift16/1 -> Data Type Conversion12/1
  Add16/1 -> Add15/2
  Delay19/1 -> Add16/2
  Data Type Conversion9/1 -> Delay15/1, Delay14/1, Delay7/1, Delay2/1, Delay13/1, Bit Concat1/1, Delay12/1, Delay17/1, Delay26/1, Delay27/1, Delay31/1, Delay32/1, Delay28/1, Delay29/1, Delay30/1, Delay33/1
  Add9/1 -> Add8/2
  Bit Shift8/1 -> Data Type Conversion10/1
  Data Type Conversion10/1 -> Delay16/1
  Add8/1 -> Add3/2
  Add3/1 -> Add2/2
  Delay1/1 -> Add2/1
  Add2/1 -> Add1/2
  Data Type Conversion5/1 -> Delay6/1
  Bit Shift7/1 -> Data Type Conversion5/1
  Delay6/1 -> Add9/1
  Delay4/1 -> Add8/1
  Bit Shift3/1 -> Data Type Conversion3/1
  Data Type Conversion3/1 -> Delay4/1
  Data Type Conversion2/1 -> Delay3/1
  Bit Shift2/1 -> Data Type Conversion2/1
  Delay3/1 -> Add3/1
  Add1/1 -> Add4/2
  Bit Shift1/1 -> Data Type Conversion1/1
  Data Type Conversion1/1 -> Delay1/1
  Data Type Conversion4/1 -> Delay5/1
  Add6/1 -> Add7/2
  Data Type Conversion7/1 -> Delay9/1
  Bit Shift5/1 -> Data Type Conversion6/1
  Delay11/1 -> Logical Operator2/2
  Chart1/3(reset_bit_counter) -> index_counter1/2(reset_bit_counter)
  Constant9/1 -> Switch4/3
  Logical Operator2/1 -> Logical Operator4/2
  Constant7/1 -> Switch3/3
  Delay10/1 -> Add6/1
  Data Type Conversion6/1 -> Delay8/1
  Add5/1 -> Add6/2
  Gain1/1 -> Scope4/3
  Switch5/1 -> Scope3/1
  Data Type Conversion8/1 -> Delay10/1
  Delay9/1 -> Add5/1
  Bit Shift6/1 -> Data Type Conversion7/1
  Clock3/1 -> Scope4/2
  Bit Shift4/1 -> Data Type Conversion4/1
  Counter Limited2/1 -> Switch3/1, Scope6/2
  Add7/1 -> Switch4/1
  Logical Operator5/1 -> Switch4/2, Gain1/1
  Delay5/1 -> Add1/1
  Logical Operator4/1 -> Switch3/2, Scope6/3, Logical Operator5/1
  Delay8/1 -> Add4/1
  index_counter1/1(index_counter) -> Chart1/1(bit_counter)
  Chart1/2(enable_bit_counter) -> index_counter1/1(enable_bit_counter)
  Switch4/1 -> Scope4/1, Data Type Conversion9/1, Chart1/2(UART_raw)
  Chart1/1(output_frame) -> Switch5/2, Scope1/1
  Constant8/1 -> Add7/1
  Clock2/1 -> Logical Operator4/1, Logical Operator2/1, Delay11/1
  Add4/1 -> Add5/2
  Bit Concat1/1 -> Switch5/1, Scope7/1
  Constant6/1 -> Switch5/3

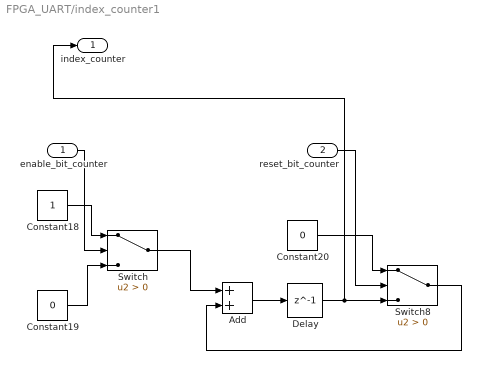
== system FPGA_UART/index_counter1 ==
  enable_bit_counter : Inport
  reset_bit_counter : Inport  Port=2
  Add : Sum  OutDataTypeStr=Inherit: Same as first input
  Constant18 : Constant  OutDataTypeStr=fixdt(0,8,0)  SampleTime=Ts
  Constant19 : Constant  Value=0  OutDataTypeStr=fixdt(0,8,0)  SampleTime=Ts
  Constant20 : Constant  Value=0  OutDataTypeStr=fixdt(0,8,0)  SampleTime=Ts
  Delay : Delay  DelayLength=1  InitialCondition=0  SampleTime=Ts
  Switch : Switch  Criteria=u2 > Threshold  SaturateOnIntegerOverflow=off  InputSameDT=off  OutDataTypeStr=Inherit: Same as first input
  Switch8 : Switch  Criteria=u2 > Threshold  SaturateOnIntegerOverflow=off  InputSameDT=off  OutDataTypeStr=Inherit: Same as first input
  index_counter : Outport
  wires:
  Constant19/1 -> Switch/3
  Switch8/1 -> Add/2
  Switch/1 -> Add/1
  Delay/1 -> index_counter/1, Switch8/3
  reset_bit_counter/1 -> Switch8/2
  Add/1 -> Delay/1
  Constant20/1 -> Switch8/1
  Constant18/1 -> Switch/1
  enable_bit_counter/1 -> Switch/2

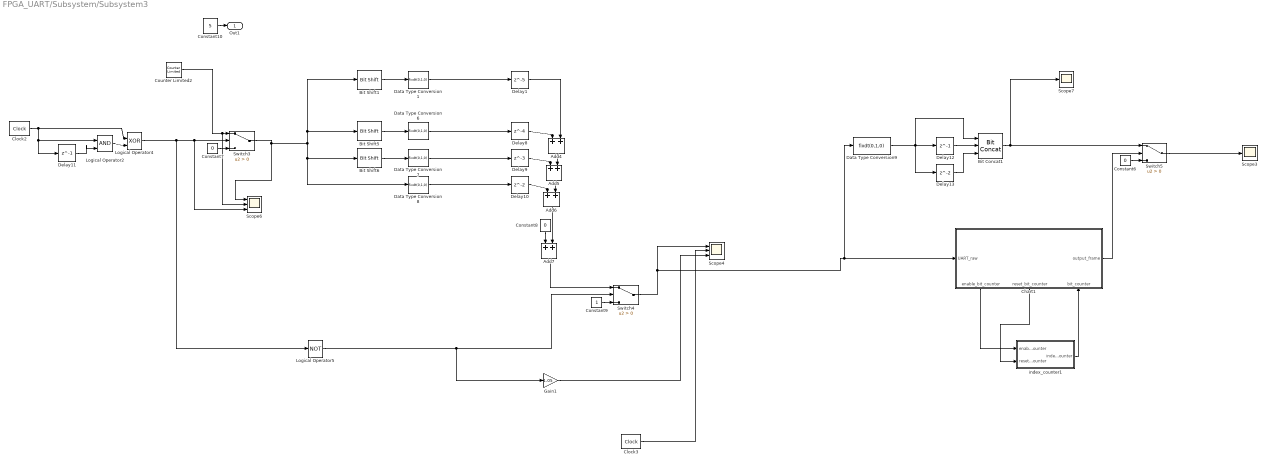
== system FPGA_UART/Subsystem/Subsystem3 ==
  Add{4..7} (4 alike) : Sum
  Bit Concat1 : hdlsllib/Logic and Bit Operations/Bit Concat  numInputs=3
  Bit Shift1 : hdlsllib/Logic and Bit Operations/Bit Shift  mode=Shift Right Logical  N=3
  Bit Shift5 : hdlsllib/Logic and Bit Operations/Bit Shift  mode=Shift Right Logical  N=2
  Bit Shift6 : hdlsllib/Logic and Bit Operations/Bit Shift  mode=Shift Right Logical  N=1
  Chart1 : Stateflow chart  TreatAsAtomicUnit=on
      settings: PortSchema="{\"entries\":[{\"content\":{\"sides\":[{\"content\":{\"connectorIds\":[\"In2\"]},\"type\":\"ConnectorPlacement.EquallySpacedRectSide\",\"uuid\":\"2ee02e2e-a069-4e33-9774-57cdf73b0390\"},{\"content\":{\"connectorIds\":[\"Out1\"],\"side\":\"RIGHT\"},\"type\":\"ConnectorPlacement.EquallySpacedRectSide\",\"uuid\":\"21aeb1e6-6c65-4c00-a9b7-a995856e37fb\"},{\"content\":{\"side\":\"TOP\"},\"type\":\"ConnectorPlacement.EquallySpacedRectSide\",\"uuid\":\"d38f9540-57bf-4030-828c-0c58160bc96c\"},{\"content\":{\"connectorIds\":[\"Out2\",\"Out3\",\"In1\"],\"side\":\"BOTTOM\"},\"type\":\"ConnectorPlacement.EquallySpacedRectSide\",\"uuid\":\"4fe203c5-9b79-43fe-8008-8789174ca3d6\"}]},\"type\":\"ConnectorPlacement.EquallySpacedConnector\",\"uuid\":\"11cdfd4e-ecb7-4173-8729-c2a9bb2b5432\"}],\"packageUris\":[\"http://schema.mathworks.com/mf0/Connector/R2020b\"],\"version\":\"1.0\"}"
  Clock2 : simulink_extras/Flip Flops/Clock  period=Ts*6
  Clock3 : simulink_extras/Flip Flops/Clock  period=Ts
  Constant10 : Constant  Value=5  OutDataTypeStr=fixdt(0,4,0)  SampleTime=Ts*5
  Constant6 : Constant  Value=0  OutDataTypeStr=fixdt(0,4,0)  SampleTime=Ts
  Constant7 : Constant  Value=0  OutDataTypeStr=fixdt(0,4,0)  SampleTime=Ts
  Constant8 : Constant  Value=0  OutDataTypeStr=fixdt(0,4,0)  SampleTime=Ts
  Constant9 : Constant  OutDataTypeStr=fixdt(0,4,0)  SampleTime=Ts
  Counter Limited2 : simulink/Sources/Counter Limited  uplimit=7  tsamp=Ts*6
  Data Type Conversion{1,6..8} (4 alike) : DataTypeConversion  OutDataTypeStr=fixdt(0,1,0)  SaturateOnIntegerOverflow=off  RndMeth=Floor
  Data Type Conversion9 : DataTypeConversion  OutDataTypeStr=fixdt(0,1,0)  RndMeth=Floor
  Delay1 : Delay  DelayLength=5  InitialCondition=0  SampleTime=Ts
  Delay10 : Delay  InitialCondition=0  SampleTime=Ts
  Delay11 : Delay  DelayLength=1  InitialCondition=0  SampleTime=Ts
  Delay12 : Delay  DelayLength=1  InitialCondition=0  SampleTime=Ts
  Delay13 : Delay  InitialCondition=0  SampleTime=Ts
  Delay8 : Delay  DelayLength=4  InitialCondition=0  SampleTime=Ts
  Delay9 : Delay  DelayLength=3  InitialCondition=0  SampleTime=Ts
  Gain1 : Gain  Gain=1.05
  Logical Operator2 : Logic  IconShape=distinctive  AllPortsSameDT=off  OutDataTypeStr=boolean
  Logical Operator4 : Logic  Operator=XOR  IconShape=distinctive  AllPortsSameDT=off  OutDataTypeStr=boolean
  Logical Operator5 : Logic  Operator=NOT  IconShape=distinctive  AllPortsSameDT=off  OutDataTypeStr=boolean
  Scope3 : Scope
  Scope4 : Scope  NumInputPorts=3
  Scope6 : Scope  NumInputPorts=3
  Scope7 : Scope
  Switch3 : Switch  Criteria=u2 > Threshold  SaturateOnIntegerOverflow=off  InputSameDT=off
  Switch4 : Switch  Criteria=u2 > Threshold  SaturateOnIntegerOverflow=off  InputSameDT=off
  Switch5 : Switch  Criteria=u2 > Threshold  OutDataTypeStr=fixdt(0,3,0)  SaturateOnIntegerOverflow=off  InputSameDT=off
  index_counter1 : Subsystem
  Out1 : Outport
  wires:
  Add6/1 -> Add7/2
  Data Type Conversion7/1 -> Delay9/1
  Bit Shift5/1 -> Data Type Conversion6/1
  Delay11/1 -> Logical Operator2/2
  Chart1/3(reset_bit_counter) -> index_counter1/2(reset_bit_counter)
  Constant9/1 -> Switch4/3
  Logical Operator2/1 -> Logical Operator4/2
  Constant7/1 -> Switch3/3
  Delay10/1 -> Add6/1
  Data Type Conversion6/1 -> Delay8/1
  Delay12/1 -> Bit Concat1/2
  Add5/1 -> Add6/2
  Gain1/1 -> Scope4/3
  Switch5/1 -> Scope3/1
  Data Type Conversion8/1 -> Delay10/1
  Delay9/1 -> Add5/1
  Delay13/1 -> Bit Concat1/3
  Bit Shift6/1 -> Data Type Conversion7/1
  Clock3/1 -> Scope4/2
  Counter Limited2/1 -> Switch3/1, Scope6/2
  Add7/1 -> Switch4/1
  Constant10/1 -> Out1/1
  Logical Operator5/1 -> Switch4/2, Gain1/1
  Logical Operator4/1 -> Switch3/2, Scope6/3, Logical Operator5/1
  Data Type Conversion9/1 -> Delay12/1, Delay13/1, Bit Concat1/1
  Delay8/1 -> Add4/1
  index_counter1/1(index_counter) -> Chart1/1(bit_counter)
  Chart1/2(enable_bit_counter) -> index_counter1/1(enable_bit_counter)
  Switch4/1 -> Scope4/1, Data Type Conversion9/1, Chart1/2(UART_raw)
  Chart1/1(output_frame) -> Switch5/2
  Constant8/1 -> Add7/1
  Clock2/1 -> Logical Operator4/1, Logical Operator2/1, Delay11/1
  Add4/1 -> Add5/2
  Bit Concat1/1 -> Scope7/1, Switch5/1
  Constant6/1 -> Switch5/3
  Delay1/1 -> Add4/2
  Switch3/1 -> Scope6/1, Bit Shift6/1, Data Type Conversion8/1, Bit Shift1/1, Bit Shift5/1
  Data Type Conversion1/1 -> Delay1/1
  Bit Shift1/1 -> Data Type Conversion1/1
